simulink model "solar_pvadd"  (R2022b)
settings: Solver=VariableStepAuto  StartTime=0.0  StopTime=10.0  RelTol=1e-3
undefined symbols (not defined in the file): D1, Delta, DiscIntNeverNeededParam, sigbuilder_block
libraries: spsSeriesRLCBranchLib x6, simulink x3, spsThreePhaseVIMeasurementLib x2, spsCurrentMeasurementLib x1, spsDiodeLib x1, spsIGBTDiodeLib x1, spsPVArrayLib x1, eeDiscretePi x1, spsFirstOrderFilterLib x1, spsThreePhaseTransformerTwoWindingsLib x1, spsThreePhaseSourceLib x1, spsUniversalBridgeLib x1
settings Model: Creator=Ideapad  LastModifiedBy=Ideapad

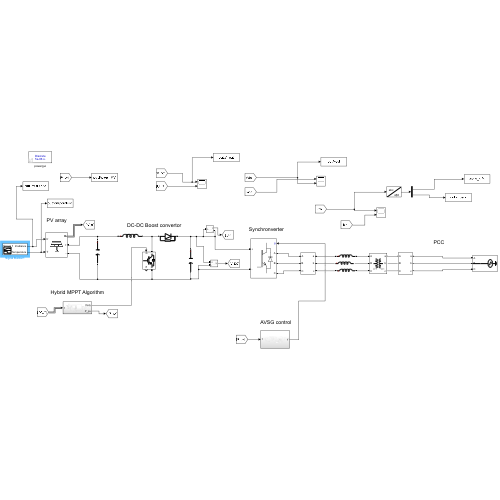
[thumbnail: Simulink's stored preview of the top-level diagram]
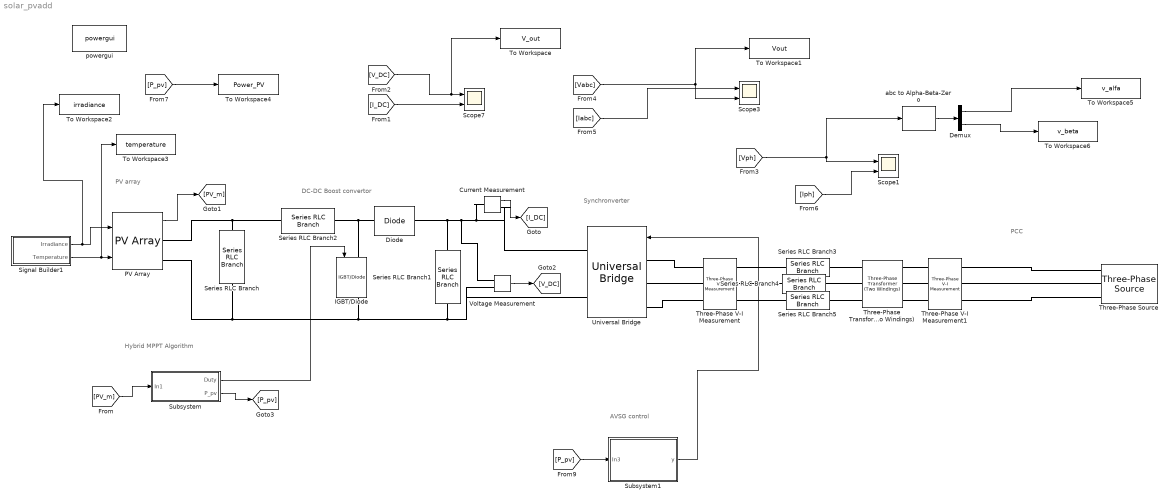
== system solar_pvadd ==
  note: Hybrid MPPT Algorithm
  note: PV array
  note: DC-DC Boost convertor
  note: AVSG control
  note: Synchronverter
  note: PCC
  Current Measurement : spsCurrentMeasurementLib/Current Measurement  PhasorSimulation=off  OutputType=Complex  PSBequivalent=0
  Demux : Demux  Outputs=2
  Diode : spsDiodeLib/Diode  Ron=0.001  Lon=0  Vf=1000.0  IC=0  UseSnubber=0  Rs=500  Cs=250e-9  Measurements=off
  IGBT/Diode : spsIGBTDiodeLib/IGBT//Diode  Ron=1e-3  Rs=1e5  Cs=inf  Measurements=on
  PV Array : spsPVArrayLib/PV Array  Npar=4  Nser=46  PlotType=array @ 1000 W/m2 & specified temperatures  S_vec="[ 1000  500  100 ]"  Temp_C_vec="[ 45 25  ]"  ModuleName=SunPower SPR-305E-WHT-D  PlotWhenSelected=off  Pm=305.226  Ncell=96  Voc=64.2  Isc=5.96  Vm=54.7  Im=5.58  beta_Voc_pc=-0.2727  alpha_Isc_pc=0.061745  beta_Voc=-0.17507  alpha_Isc=0.00368  IL=5.9657  I0=6.3076e-12  nI=0.94489  Rsh=393.2054  Rs=0.37428  RobustModel=off  RobustCellTemperature=313.3991  BAL=on  Tc=1e-6  Tfilter=5e-5
  Scope1 : Scope  NumInputPorts=2
  Scope3 : Scope  NumInputPorts=2
  Scope7 : Scope  NumInputPorts=2
  Series RLC Branch : spsSeriesRLCBranchLib/Series RLC Branch  LConnTagsString=__new0  RConnTagsString=__new0  BranchType=C  Resistance=1  Inductance=1e-3  SetiL0=off  InitialCurrent=0  Capacitance=83e-6  Setx0=off  InitialVoltage=0  Measurements=None
  Series RLC Branch1 : spsSeriesRLCBranchLib/Series RLC Branch  LConnTagsString=__new0  RConnTagsString=__new0  BranchType=C  Resistance=1  Inductance=1e-3  SetiL0=off  InitialCurrent=0  Capacitance=83e-6  Setx0=off  InitialVoltage=0  Measurements=None
  Series RLC Branch2 : spsSeriesRLCBranchLib/Series RLC Branch  LConnTagsString=__new0  RConnTagsString=__new0  BranchType=L  Resistance=1  Inductance=0.25  SetiL0=off  InitialCurrent=0  Capacitance=1e-6  Setx0=off  InitialVoltage=0  Measurements=None
  Series RLC Branch3 : spsSeriesRLCBranchLib/Series RLC Branch  LConnTagsString=__new0  RConnTagsString=__new0  BranchType=L  Resistance=1  Inductance=0.90e-3  SetiL0=off  InitialCurrent=0  Capacitance=1e-6  Setx0=off  InitialVoltage=0  Measurements=None
  Series RLC Branch4 : spsSeriesRLCBranchLib/Series RLC Branch  LConnTagsString=__new0  RConnTagsString=__new0  BranchType=L  Resistance=1  Inductance=0.90e-3  SetiL0=off  InitialCurrent=0  Capacitance=1e-6  Setx0=off  InitialVoltage=0  Measurements=None
  Series RLC Branch5 : spsSeriesRLCBranchLib/Series RLC Branch  LConnTagsString=__new0  RConnTagsString=__new0  BranchType=L  Resistance=1  Inductance=0.90e-3  SetiL0=off  InitialCurrent=0  Capacitance=1e-6  Setx0=off  InitialVoltage=0  Measurements=None
  Signal Builder1 : Subsystem  Tag=STV Subsys  LoadFcn=sigbuilder_block('load');  StartFcn=sigbuilder_block('start');  StopFcn=sigbuilder_block('stop');  ClipboardFcn=sigbuilder_block('clipboard');  mask(Sigbuilder block){tuvar=[0:10]}
      mask help: Simulink:masks:SigbuilderBlock_MD
      mask init:
      | if ~strcmp(get_param(bdroot(gcbh),'SimulationStatus'),'stopped') tuvar = sigbuilder_block('maskInit'); end
      settings: CopyFcn=sigbuilder_block('copy');  DeleteFcn=sigbuilder_block('delete');  ModelCloseFcn=sigbuilder_block('modelClose');  PreSaveFcn=sigbuilder_block('preSave');  PauseFcn=sigbuilder_block('pause');  ContinueFcn=sigbuilder_block('continue');  NameChangeFcn=sigbuilder_block('namechange');  OpenFcn=sigbuilder_block('open',[0 36 1152 555.6 ]);  CloseFcn=sigbuilder_block('close');
      mask Display: plot(0, 0, 100, 100,[2, 2, 32, 32, 2], [68, 8, 8, 68, 68],[32, 2], [38, 38], [32, 19, 2],[53, 60, 44], [32, 17, 17, 2],[16, 16, 31, 31]);txt = getActiveGroup(gcbh);text(2, 100, txt,'verticalAlignment', 'top');
  Subsystem : Subsystem
  Subsystem1 : Subsystem
  Three-Phase Transformer (Two Windings) : spsThreePhaseTransformerTwoWindingsLib/Three-Phase Transformer (Two Windings)  Winding1Connection=Delta (D1)  Winding2Connection=Delta (D1)  CoreType=Three single-phase transformers  SetSaturation=off  Hysteresis=off  DataFile='hysteresis'  SetInitialFlux=off  Measurements=None  UNITS=pu  NominalPower=[ 25e3 , 50 ]  Winding1=[ 2.9e3 , 0.002 , 0.08 ]  Winding2=[ 25e3 , 0.002 , 0.08 ]  Rm=500  Lm=500  L0=0.5  Saturation=[ 0,0 ; 0.0024,1.2 ; 1.0,1.52 ]  InitialFluxes=[ 0.8 , -0.8 , 0.7 ]  BreakLoop=off  DiscreteSolver=Trapezoidal iterative  DataType=off  TransfoNumber=1
  Three-Phase V-I Measurement : spsThreePhaseVIMeasurementLib/Three-Phase V-I Measurement  VoltageMeasurement=phase-to-phase  SetLabelV=on  LabelV=Vabc  Vpu=off  VpuLL=off  CurrentMeasurement=yes  SetLabelI=on  LabelI=Iabc  Ipu=off  Pbase=100e6  Vbase=500e3  OutputType=Complex  PhasorSimulation=off  PSBequivalent=0
  Three-Phase V-I Measurement1 : spsThreePhaseVIMeasurementLib/Three-Phase V-I Measurement  VoltageMeasurement=phase-to-phase  SetLabelV=on  LabelV=Vph  Vpu=off  VpuLL=off  CurrentMeasurement=yes  SetLabelI=on  LabelI=Iph  Ipu=off  Pbase=100e6  Vbase=500e3  OutputType=Complex  PhasorSimulation=off  PSBequivalent=0
  Three-Phase Source : spsThreePhaseSourceLib/Three-Phase Source  InternalConnection=Yg  VoltagePhases=on  Voltage=25e3  PhaseAngle=0  Voltage_phases=[25e3 25e3 25e3]/sqrt(3)  PhaseAngles_phases=[0 -120 +120]  Frequency=50  NonIdealSource=off  SpecifyImpedance=off  Resistance=0.8929  Inductance=16.58e-3  ShortCircuitLevel=100e6  BaseVoltage=25e3  XRratio=7  BusType=PV  Pref=10e3  Qref=0  Prefabc=[10e3, 10e3, 10e3]  Qrefabc=[0, 0, 0]  Qmin=-inf  Qmax=inf
  To Workspace : ToWorkspace  VariableName=V_out  SaveFormat=Structure With Time  SampleTime=-1
  To Workspace1 : ToWorkspace  VariableName=Vout  SaveFormat=Structure With Time  SampleTime=-1
  To Workspace2 : ToWorkspace  VariableName=irradiance  SaveFormat=Timeseries  SampleTime=-1
  To Workspace3 : ToWorkspace  VariableName=temperature  SaveFormat=Timeseries  SampleTime=-1
  To Workspace4 : ToWorkspace  VariableName=Power_PV  SaveFormat=Structure With Time  SampleTime=-1
  To Workspace5 : ToWorkspace  VariableName=v_alfa  SaveFormat=Structure With Time  SampleTime=-1
  To Workspace6 : ToWorkspace  VariableName=v_beta  SaveFormat=Structure With Time  SampleTime=-1
  Universal Bridge : spsUniversalBridgeLib/Universal Bridge  Arms=3  SnubberResistance=1e3  SnubberCapacitance=1e-6  Device=IGBT / Diodes  Ron=1e-3  Lon=0  ForwardVoltages="[  0  0  ]"  ForwardVoltage=0  GTOparameters=[ 10e-6 , 20e-6 ]  IGBTparameters=[ 1e-6 , 2e-6 ]  Measurements=Device voltages  Measurements_2=None  converterType=Rectifier
  Voltage Measurement : spsVoltageMeasurementLib/Voltage Measurement  PhasorSimulation=off  OutputType=Complex  PSBequivalent=0
  abc to Alpha-Beta-Zero : spsabctoAlphaBetaZeroLib/abc to Alpha-Beta-Zero
  powergui : sps_lib/powergui  Priority=1  SimulationMode=Discrete  SampleTime=5e-6  frequency=60  Iterations=50  frequencyindice=50  Pbase=100e6  ErrMax=1e-4  UnitsV=kV  UnitsW=MW  buscounter=0  FunctionMessages=off  echomessages=off  EnableUseOfTLC=off  CurrentSourceSwitches=off  DisableSnubberDevices=off  DisableRonSwitches=off  DisableVfSwitches=off  DisplayEquations=off  AutomaticDiscreteSolvers=off  SolverType=Tustin/Backward Euler (TBE)  Interpol=off  ExternalGateDelay=off  methode=off  Ts=100  x0status=blocks  SPID=on  SwTol=0  HookPort=off  NonlinearTolerance=1e-4  nMaxIteration=100  ContinueOnMaxIteration=off  RestoreLinks=warning  ResistiveCurrentMeasurement=off  Frange=[0:2:500]  Ylog=off  Xlog=on  ShowGrid=off  save=off  variable=ZData  structure=0  ZoomFFT=off  StartTime=0.0  cycles=1  DisplayStyle=1  fundamental=60  FreqAxis=off  MaxFrequency=1000  frequencyindicesteady=1  RmsSteady=1  display=off
  wires:
  Voltage Measurement/1 -> [V_DC]
  PV Array/1 -> [PV_m]
  [PV_m] -> Subsystem/1(In1)
  Current Measurement/1 -> [I_DC]
  Signal Builder1/1(Irradiance) -> To Workspace2/1, PV Array/1
  Signal Builder1/2(Temperature) -> To Workspace3/1, PV Array/2
  Subsystem/1(Duty) -> IGBT/Diode/1
  Subsystem/2(P_pv) -> [P_pv]
  Subsystem1/1(y) -> Universal Bridge/1
  [P_pv] -> Subsystem1/1(In3)
  [Vabc] -> To Workspace1/1, Scope3/2
  [V_DC] -> To Workspace/1, Scope7/1
  [I_DC] -> Scope7/2
  [Vph] -> Scope1/1, abc to Alpha-Beta-Zero/1
  [P_pv] -> To Workspace4/1
  abc to Alpha-Beta-Zero/1 -> Demux/1
  Demux/1 -> To Workspace5/1
  Demux/2 -> To Workspace6/1
  [Iabc] -> Scope3/1
  [Iph] -> Scope1/2
  connections:
  PV Array/RConn1 -- Series RLC Branch/LConn1 -- Series RLC Branch2/LConn1
  Diode/LConn1 -- Series RLC Branch2/RConn1 -- IGBT/Diode/LConn1
  Diode/RConn1 -- Current Measurement/RConn1 -- Universal Bridge/RConn1 -- Current Measurement/LConn1 -- Voltage Measurement/LConn1 -- Series RLC Branch1/LConn1
  Series RLC Branch1/RConn1 -- Voltage Measurement/LConn2 -- Universal Bridge/RConn2 -- Series RLC Branch/RConn1 -- PV Array/RConn2 -- IGBT/Diode/RConn1
  Three-Phase V-I Measurement/LConn1 -- Universal Bridge/LConn1
  Three-Phase V-I Measurement/LConn2 -- Universal Bridge/LConn2
  Universal Bridge/LConn3 -- Three-Phase V-I Measurement/LConn3
  Series RLC Branch3/LConn1 -- Three-Phase V-I Measurement/RConn1
  Series RLC Branch4/LConn1 -- Three-Phase V-I Measurement/RConn2
  Series RLC Branch5/LConn1 -- Three-Phase V-I Measurement/RConn3
  Series RLC Branch3/RConn1 -- Three-Phase Transformer (Two Windings)/LConn1
  Series RLC Branch4/RConn1 -- Three-Phase Transformer (Two Windings)/LConn2
  Series RLC Branch5/RConn1 -- Three-Phase Transformer (Two Windings)/LConn3
  Three-Phase Transformer (Two Windings)/RConn1 -- Three-Phase V-I Measurement1/LConn1
  Three-Phase Transformer (Two Windings)/RConn2 -- Three-Phase V-I Measurement1/LConn2
  Three-Phase Transformer (Two Windings)/RConn3 -- Three-Phase V-I Measurement1/LConn3
  Three-Phase V-I Measurement1/RConn1 -- Three-Phase Source/RConn1
  Three-Phase V-I Measurement1/RConn2 -- Three-Phase Source/RConn2
  Three-Phase V-I Measurement1/RConn3 -- Three-Phase Source/RConn3

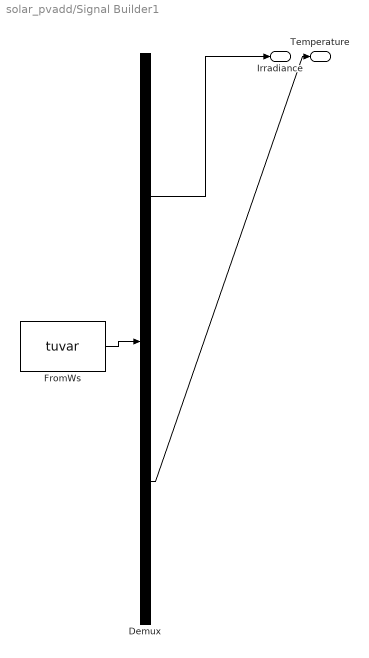
== system solar_pvadd/Signal Builder1 ==
  Demux : Demux  Tag=STV Demux  Outputs=2
      settings: DisplayOption=none
  FromWs : FromWorkspace  Tag=STV FromWs  VariableName=tuvar
      SigBuilderData=|
      | common.afterFinalStr = 'Extrapolate'
      | common.sampleTime = 0
      | dataSet.timeRange = [0 10]
      | dataSet.name = 'Group 1'
      | sbobj.Groups.Name = 'Group 1'
      | sbobj.Groups.Signals(1).Name = 'Irradiance'
      | sbobj.Groups.Signals(1).XData = [0 2 4 6 8 10]
      | sbobj.Groups.Signals(1).YData = [1000 800 600 1000 900 1000]
      | sbobj.Groups.Signals(2).Name = 'Temperature'
      | sbobj.Groups.Signals(2).XData = [0 2 4 6 8 10]
      | sbobj.Groups.Signals(2).YData = [25 30 35 40 30 25]
  Irradiance : Outport  Tag=STV Outport
  Temperature : Outport  Tag=STV Outport  Port=2
  wires:
  Demux/1 -> Irradiance/1
  FromWs/1 -> Demux/1
  Demux/2 -> Temperature/1

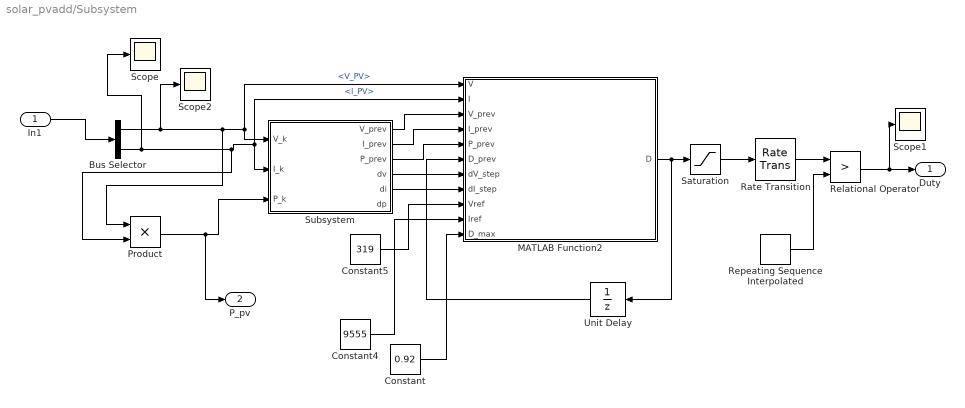
== system solar_pvadd/Subsystem ==
  In1 : Inport
  Bus Selector : BusSelector  OutputSignals=V_PV,I_PV
  Constant : Constant  Value=0.92
  Constant4 : Constant  Value=9555
  Constant5 : Constant  Value=319
  MATLAB Function2 : MATLAB Function  TreatAsAtomicUnit=on
  Product : Product
  Rate Transition : RateTransition  OutPortSampleTime=50e-6
  Relational Operator : RelationalOperator  Operator=>  OutDataTypeStr=boolean  RndMeth=Simplest  InputSameDT=off
  Repeating Sequence Interpolated : simulink/Sources/Repeating Sequence Interpolated  OutValues=[0 1].'  TimeValues=[0 5e-5].'  LookUpMeth=Interpolation-Use End Values  tsamp=5e-5  OutMin=[]  OutMax=[]  OutDataTypeStr=double  OutputDataTypeScalingMode=double  OutDataType=fixdt(0,8)  OutScaling=2^-10
  Saturation : Saturate  UpperLimit=0.90  LowerLimit=0.02
  Scope : Scope
  Scope1 : Scope
  Scope2 : Scope
  Subsystem : Subsystem
  Unit Delay : UnitDelay  SampleTime=0.01  HasFrameUpgradeWarning=on
  Duty : Outport
  P_pv : Outport  Port=2
  wires:
  In1/1 -> Bus Selector/1
  Bus Selector/1 -> Scope2/1, Product/1, MATLAB Function2/1(V), Subsystem/1(V_k)  "<V_PV>"
  Bus Selector/2 -> Scope/1, Product/2, MATLAB Function2/2(I), Subsystem/2(I_k)  "<I_PV>"
  Product/1 -> P_pv/1, Subsystem/3(P_k)
  Subsystem/4(dv) -> MATLAB Function2/7(dV_step)
  Subsystem/5(di) -> MATLAB Function2/8(dI_step)
  Subsystem/1(V_prev) -> MATLAB Function2/3(V_prev)
  Subsystem/2(I_prev) -> MATLAB Function2/4(I_prev)
  Subsystem/3(P_prev) -> MATLAB Function2/5(P_prev)
  Unit Delay/1 -> MATLAB Function2/6(D_prev)
  Constant5/1 -> MATLAB Function2/9(Vref)
  Constant4/1 -> MATLAB Function2/10(Iref)
  Constant/1 -> MATLAB Function2/11(D_max)
  MATLAB Function2/1(D) -> Unit Delay/1, Saturation/1
  Saturation/1 -> Rate Transition/1
  Rate Transition/1 -> Relational Operator/1
  Repeating Sequence Interpolated/1 -> Relational Operator/2
  Relational Operator/1 -> Scope1/1, Duty/1

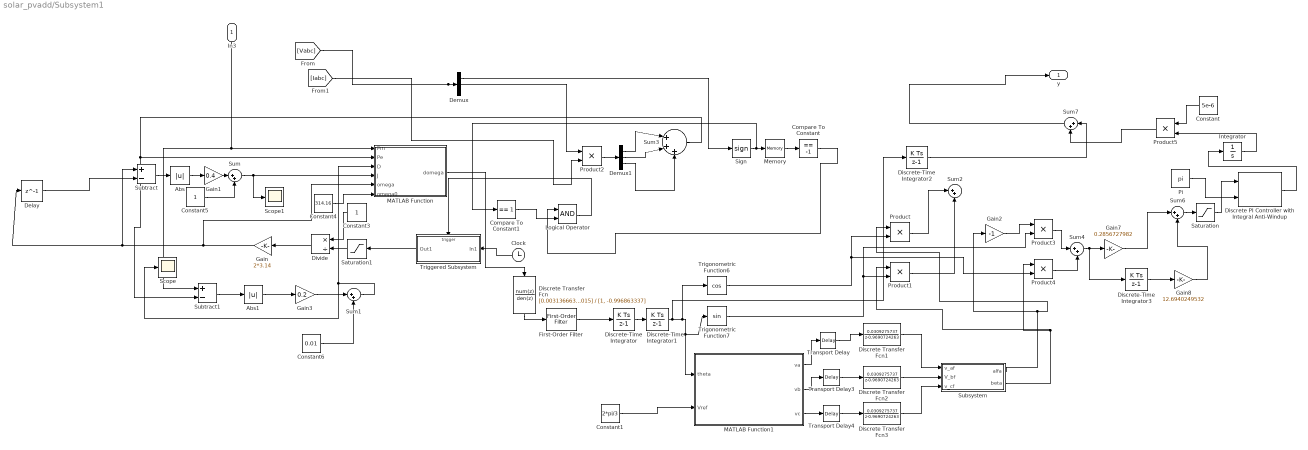
== system solar_pvadd/Subsystem1 ==
  In3 : Inport
  Abs : Abs  SaturateOnIntegerOverflow=off
  Abs1 : Abs  SaturateOnIntegerOverflow=off
  Clock : Clock
  Compare To Constant : simulink/Logic and Bit Operations/Compare To Constant  relop===  const=-1  OutDataTypeStr=boolean
  Compare To Constant1 : simulink/Logic and Bit Operations/Compare To Constant  relop===  const=1  OutDataTypeStr=boolean
  Constant : Constant  Value=5e-6
  Constant1 : Constant  Value=2*pi/3
  Constant3 : Constant
  Constant4 : Constant  Value=314.16  SampleTime=5e-6
  Constant5 : Constant
  Constant6 : Constant  Value=0.01
  Delay : Delay  DelayLength=1  InitialCondition=0
  Demux : Demux  Outputs=3
  Demux1 : Demux  Outputs=3
  Discrete Transfer Fcn : DiscreteTransferFcn  Numerator=[0.003136663015]  Denominator=[1, -0.996863337]  SampleTime=5e-6
  Discrete Transfer Fcn1 : DiscreteTransferFcn  Numerator=[0.0309275737]  Denominator=[1, -0.9690724263]  SampleTime=5e-6
  Discrete Transfer Fcn2 : DiscreteTransferFcn  Numerator=[0.0309275737]  Denominator=[1, -0.9690724263]  SampleTime=5e-6
  Discrete Transfer Fcn3 : DiscreteTransferFcn  Numerator=[0.0309275737]  Denominator=[1, -0.9690724263]  SampleTime=5e-6
  Discrete PI Controller with Integral Anti-Windup : eeDiscretePi/Discrete PI Controller with Integral Anti-Windup  Kp=1  Ki=1  x0=0  B=5  A=-5  Ts=-1
      settings: LibrarySourceBlock=|
      | ee_sl_lib/General Control/Discrete PI Controller
      | with Integral Anti-Windup
  Discrete-Time Integrator : DiscreteIntegrator  gainval=5e-6  InitialCondition=2*pi*50  SampleTime=5e-6  ICPrevOutput=DiscIntNeverNeededParam  ICPrevScaledInput=DiscIntNeverNeededParam
  Discrete-Time Integrator1 : DiscreteIntegrator  gainval=5e-6  SampleTime=5e-6  ICPrevOutput=DiscIntNeverNeededParam  ICPrevScaledInput=DiscIntNeverNeededParam
  Discrete-Time Integrator2 : DiscreteIntegrator  SampleTime=-1  ICPrevOutput=DiscIntNeverNeededParam  ICPrevScaledInput=DiscIntNeverNeededParam
  Discrete-Time Integrator3 : DiscreteIntegrator  SampleTime=5e-6  ICPrevOutput=DiscIntNeverNeededParam  ICPrevScaledInput=DiscIntNeverNeededParam
  Divide : Product  Inputs=*/
  First-Order Filter : spsFirstOrderFilterLib/First-Order Filter  FilterType=Lowpass  Tc=5e-6  Ts=1  Initialize=on  Vac_Init=[0, 0, 50]  Vdc_Init=0  PlotResponse=off  FreqRange="[0,  200,  1]"
  Gain : Gain  Gain=2*3.14
  Gain1 : Gain  Gain=0.4
  Gain2 : Gain  Gain=-1
  Gain3 : Gain  Gain=0.2
  Gain7 : Gain  Gain=0.2856727982
  Gain8 : Gain  Gain=12.6940249532
  Integrator : Integrator
  Logical Operator : Logic  AllPortsSameDT=off  OutDataTypeStr=boolean
  MATLAB Function : MATLAB Function  TreatAsAtomicUnit=on
  MATLAB Function1 : MATLAB Function  TreatAsAtomicUnit=on
  Memory : Memory
  Pi : Constant  Value=pi  OutDataTypeStr=Inherit: Inherit via back propagation
  Product{,1..5} (6 alike) : Product
  Saturation : Saturate  UpperLimit=+2*3.14*5  LowerLimit=-2*3.14*5
  Saturation1 : Saturate  UpperLimit=1e3  LowerLimit=1e-6
  Scope : Scope
  Scope1 : Scope
  Sign : Signum
  Subsystem : Subsystem
  Subtract : Sum  Inputs=+-
  Subtract1 : Sum  Inputs=+-
  Sum{,1..2,4,6..7} (6 alike) : Sum  Inputs=|++
  Sum3 : Sum  Inputs=|+++
  Transport Delay : TransportDelay  DelayTime=1.67e-3  InitialOutput=1
  Transport Delay3 : TransportDelay  DelayTime=1.67e-3  InitialOutput=1
  Transport Delay4 : TransportDelay  DelayTime=1.67e-3  InitialOutput=1
  Triggered Subsystem : Subsystem  TreatAsAtomicUnit=on
  Trigonometric Function6 : Trigonometry  Operator=cos
  Trigonometric Function7 : Trigonometry
  y : Outport
  wires:
  Sum/1 -> Scope1/1, MATLAB Function/4(J)
  Delay/1 -> Subtract/2
  MATLAB Function/1(domega) -> Discrete Transfer Fcn/1
  Constant3/1 -> Divide/1
  Compare To Constant/1 -> Logical Operator/1
  Constant5/1 -> Sum/2
  Constant6/1 -> Sum1/2
  Logical Operator/1 -> Triggered Subsystem/Trigger
  Sum1/1 -> Scope/1, MATLAB Function/3(D)
  Saturation1/1 -> Divide/2
  Demux1/2 -> Sum3/2
  Product2/1 -> Demux1/1
  Demux1/1 -> Sum3/1
  Compare To Constant1/1 -> Logical Operator/2
  Clock/1 -> Triggered Subsystem/1(In1)
  Subtract1/1 -> Abs1/1
  Abs1/1 -> Gain3/1
  Gain1/1 -> Sum/1
  Divide/1 -> Gain/1
  Triggered Subsystem/1(Out1) -> Saturation1/1
  Gain3/1 -> Sum1/1
  Sum3/1 -> Subtract1/2, MATLAB Function/2(Pe)
  Memory/1 -> Compare To Constant/1
  Constant4/1 -> MATLAB Function/6(omega0)
  Demux/1 -> Sign/1
  Sign/1 -> Compare To Constant1/1, Memory/1
  Subtract/1 -> Abs/1
  Gain/1 -> Subtract/1, Delay/1, MATLAB Function/5(omega)
  In3/1 -> Subtract1/1, MATLAB Function/1(Pm)
  Demux1/3 -> Sum3/3
  Abs/1 -> Gain1/1
  Discrete Transfer Fcn/1 -> First-Order Filter/1
  Discrete-Time Integrator/1 -> Discrete-Time Integrator1/1
  Constant1/1 -> MATLAB Function1/2(Vref)
  MATLAB Function1/1(va) -> Transport Delay/1
  MATLAB Function1/3(vc) -> Transport Delay4/1
  Trigonometric Function6/1 -> Product/2, Product4/2
  Trigonometric Function7/1 -> Product3/2, Product1/2
  Subsystem/1(alfa) -> Product/1, Gain2/1
  Subsystem/2(beta) -> Product4/1, Product1/1
  Product/1 -> Sum2/1
  Product1/1 -> Sum2/2
  Gain2/1 -> Product3/1
  Product3/1 -> Sum4/1
  Product4/1 -> Sum4/2
  Discrete Transfer Fcn1/1 -> Subsystem/1(v_af)
  Discrete Transfer Fcn2/1 -> Subsystem/2(V_bf)
  Discrete Transfer Fcn3/1 -> Subsystem/3(v_cf)
  Sum4/1 -> Discrete-Time Integrator3/1, Gain7/1
  Sum6/1 -> Saturation/1
  Saturation/1 -> Discrete PI Controller with Integral Anti-Windup/1
  Pi/1 -> Discrete PI Controller with Integral Anti-Windup/2
  Discrete PI Controller with Integral Anti-Windup/1 -> Integrator/1
  Integrator/1 -> Product5/2
  Constant/1 -> Product5/1
  Discrete-Time Integrator2/1 -> Sum7/1
  Product5/1 -> Sum7/2
  Discrete-Time Integrator3/1 -> Gain8/1
  Gain7/1 -> Sum6/1
  Gain8/1 -> Sum6/2
  Sum7/1 -> y/1
  First-Order Filter/1 -> Discrete-Time Integrator/1
  [Vabc] -> Demux/1, Product2/1
  [Iabc] -> Product2/2
  Discrete-Time Integrator1/1 -> Discrete-Time Integrator2/1, Trigonometric Function6/1, MATLAB Function1/1(theta), Trigonometric Function7/1
  Transport Delay/1 -> Discrete Transfer Fcn1/1
  MATLAB Function1/2(vb) -> Transport Delay3/1
  Transport Delay3/1 -> Discrete Transfer Fcn2/1
  Transport Delay4/1 -> Discrete Transfer Fcn3/1

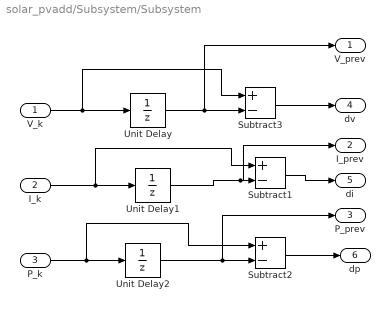
== system solar_pvadd/Subsystem/Subsystem ==
  V_k : Inport
  I_k : Inport  Port=2
  P_k : Inport  Port=3
  Subtract1 : Sum  Inputs=+-
  Subtract2 : Sum  Inputs=+-
  Subtract3 : Sum  Inputs=+-
  Unit Delay : UnitDelay  SampleTime=0.01  HasFrameUpgradeWarning=on
  Unit Delay1 : UnitDelay  SampleTime=0.01  HasFrameUpgradeWarning=on
  Unit Delay2 : UnitDelay  SampleTime=0.01  HasFrameUpgradeWarning=on
  V_prev : Outport
  I_prev : Outport  Port=2
  P_prev : Outport  Port=3
  dv : Outport  Port=4
  di : Outport  Port=5
  dp : Outport  Port=6
  wires:
  V_k/1 -> Unit Delay/1, Subtract3/1
  I_k/1 -> Unit Delay1/1, Subtract1/1
  P_k/1 -> Unit Delay2/1, Subtract2/1
  Subtract1/1 -> di/1
  Subtract2/1 -> dp/1
  Unit Delay/1 -> V_prev/1, Subtract3/2
  Subtract3/1 -> dv/1
  Unit Delay1/1 -> I_prev/1, Subtract1/2
  Unit Delay2/1 -> P_prev/1, Subtract2/2

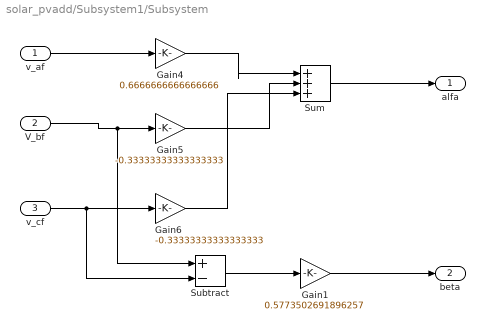
== system solar_pvadd/Subsystem1/Subsystem ==
  v_af : Inport
  V_bf : Inport  Port=2
  v_cf : Inport  Port=3
  Gain1 : Gain  Gain=0.5773502691896257
  Gain4 : Gain  Gain=0.6666666666666666
  Gain5 : Gain  Gain=-0.33333333333333333
  Gain6 : Gain  Gain=-0.33333333333333333
  Subtract : Sum  Inputs=+-
  Sum : Sum  Inputs=|+++
  alfa : Outport
  beta : Outport  Port=2
  wires:
  v_af/1 -> Gain4/1
  V_bf/1 -> Subtract/1, Gain5/1
  v_cf/1 -> Subtract/2, Gain6/1
  Gain4/1 -> Sum/1
  Gain5/1 -> Sum/2
  Gain6/1 -> Sum/3
  Sum/1 -> alfa/1
  Subtract/1 -> Gain1/1
  Gain1/1 -> beta/1

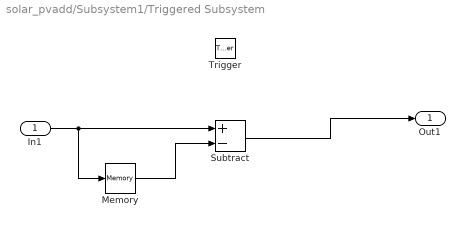
== system solar_pvadd/Subsystem1/Triggered Subsystem ==
  In1 : Inport
  Trigger : TriggerPort  VariantControl=(inherit)
  Memory : Memory  InitialCondition=-1  InheritSampleTime=on
  Subtract : Sum  Inputs=+-
  Out1 : Outport
  wires:
  In1/1 -> Subtract/1, Memory/1
  Memory/1 -> Subtract/2
  Subtract/1 -> Out1/1

== matlab function solar_pvadd/Subsystem1/MATLAB Function ==
  data: Pm input; domega output; Pe input; D input; J input; omega input; omega0 input
function domega = swing(Pm, Pe, D, J, omega, omega0)
domega = (Pm - Pe - D * (omega - omega0)) / J;
end

== matlab function solar_pvadd/Subsystem1/MATLAB Function1 ==
  data: theta input; va output; Vref input; vb output; vc output
function [va,vb,vc] = threePhaseRefs(theta, Vref)
% theta: scalar theta_avsg (rad)
% Vref:  scalar amplitude
vb = Vref * sin(theta - 2*pi/3);
vc = Vref * sin(theta + 2*pi/3);
va = Vref * sin(theta);
end

== matlab function solar_pvadd/Subsystem/MATLAB Function2 ==
  data: V input; D output; I input; V_prev input; I_prev input; P_prev input; D_prev input; dV_step input; dI_step input; Vref input; Iref input; D_max input
function D = Hybrid_MPPT(V, I, V_prev, I_prev, P_prev, D_prev, dV_step, dI_step, Vref, Iref, D_max)
% Hybrid MPPT using VPA + CPA + ACA with weighting

% 1) Power calculation
P = V * I;

% 2) Voltage Perturbation Algorithm (VPA)
dV = V - V_prev;
dP = P - P_prev;

if dP > 0
    if dV > 0
        dVpa = -dV_step;  % Move towards MPP
    else
        dVpa = dV_step;
    end
else
    if dV > 0
        dVpa = dV_step;   % Move away from wrong side
    else
        dVpa = -dV_step;
    end
end

% 3) Current Perturbation Algorithm (CPA)
dI = I - I_prev;

if dP > 0
    if dI > 0
        dCpa = -dI_step;
    else
        dCpa = dI_step;
    end
else
    if dI > 0
        dCpa = dI_step;
    else
        dCpa = -dI_step;
    end
end

% 4) Adaptive Control Algorithm (ACA)
Vmpp_ratio = V / Vref;
Impp_ratio = I / Iref;

if Vmpp_ratio > 0.8 && Impp_ratio > 0.8
    dAca = -0.001; % step down duty
else
    dAca = 0.001;  % step up duty
end

% 5) Weighted combination
D = D_prev + (0.4 * dVpa) + (0.3 * dCpa) + (0.3 * dAca);

% 6) Limit duty cycle
D = max(0, min(D, D_max));

end
